simulink library "simpower_extensions_1"  (Simulink 7.4)
settings: Solver=ode45  SolverMode=SingleTasking  StartTime=0.0  StopTime=10.0  RelTol=1e-3
values from neighbouring files (symbols this model uses):
  Av = 10^(Gdb/20)    (= 6.3095734448)    [series_shunt_2c.m]
undefined symbols (not defined in the file or in its folder): f1, f2, Fs, get, magnitude, One, sided, Two
libraries: powerlib x71, dspindex x36, dsparch4 x22, dspsigops x18, dspbuff3 x12, dspxfrm3 x12, dsparch3 x12, dspsnks4 x6, dspmtrx3 x6, simpower_extensions_1 x1, simulink x1, simulink_extras x1
(part 1 of 3)
settings Model: Creator=Dick Benson  LastModifiedBy=Dick  ModifiedHistory=1st cut at EE circuit library.

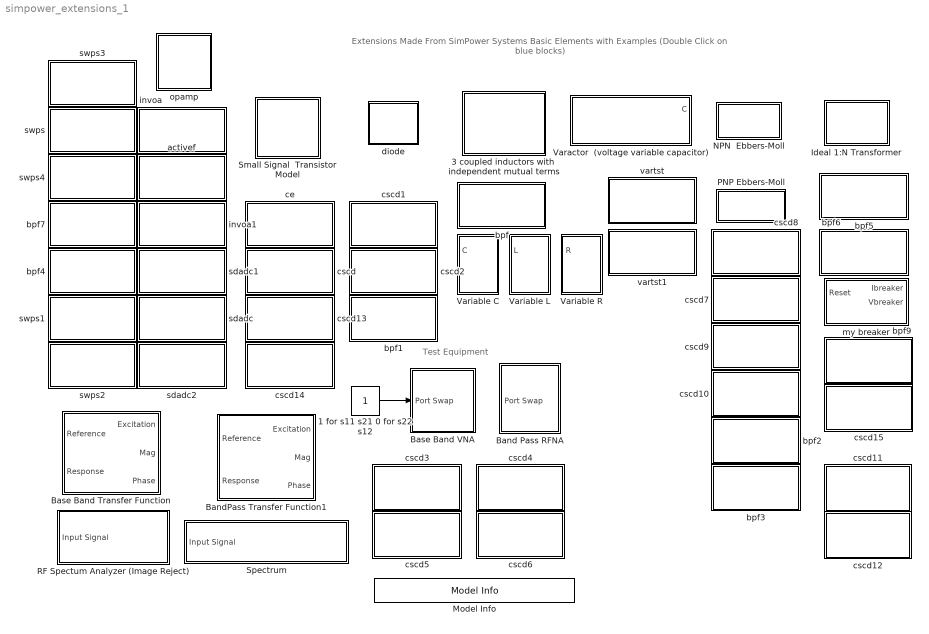
== system simpower_extensions_1 ==
  note: Extensions Made From SimPower Systems Basic Elements
      | with Examples (Double Click on blue blocks)
  note: Test Equipment
  1 for s11 s21 0 for s22 s12 : Constant  OutDataType=fixdt(1, 16)  OutScaling=2^0
  3 coupled inductors with  independent mutual terms : Subsystem  mask{L1=1e-6, L2=1e-6, L3=1e-6, M12=0.1e-6, M23=0.1e-6, M13=1e-8}
      mask prompts: L1 "L1="; L2 "L2="; L3 "L3="; M12 "M12="; M23 "M23="; M13 "M13="
  Band Pass RFNA : Subsystem  Description=Spectrum Analyzer  mask{Fc=75e6, BW=20e6, Frame_Size=512}
      mask prompts: Fc "Center Freq"; BW "Bandwidth"; Frame_Size "FFT SIze (256,512,1024 etc)"
  BandPass Transfer Function1 : Subsystem  Description=Spectrum Analyzer  mask{BW=40e6, Fc=100e6, NFFT=1024, Avg_fac=100}
      mask prompts: BW "Bandwidth"; Fc "Center Freq"; NFFT "FFT Length (power of 2)"; Avg_fac "Averaging Factor (>=1)"
  Base Band Transfer Function : Subsystem  Description=Spectrum Analyzer  mask{BW=100e6, NFFT=1024, Avg_fac=100}
      mask prompts: BW "Bandwidth"; NFFT "FFT Length (power of 2)"; Avg_fac "Averaging Factor (>=1)"
  Base Band VNA : Subsystem  Description=Spectrum Analyzer  mask{BW=2e8, Frame_Size=512}
      mask prompts: BW "Bandwidth"; Frame_Size "FFT SIze (256,512,1024 etc)"
  Ideal 1:N Transformer : Subsystem  mask{N=10}
      mask prompts: N "Turns Ratio Secondary/Primary"
  Model Info : simulink/Model-Wide Utilities/Model Info  SystemSampleTime=-1  InitialBlockCM=None  BlockCM=None  Frame=on  DisplayStringWithTags=Copywrite 2005-2011 The MathWorks, Inc.  HorizontalTextAlignment=Center  LeftAlignmentValue=0.5  SourceBlockDiagram=simpower_extensions_1  TagMaxNumber=20
  "NPN  Ebbers-Moll " : Subsystem  mask{Beta=100, IEs=1e-8;, ICs=1e-8;, Ro=1e5, Cbc=5e-12, Cbe=50e-12, Rbb=100}
      mask init:
      | k = 1.38e-23;
      | q = 1.6e-19;
      | T = 290;
      | Vt = k*T/q;
  PNP Ebbers-Moll : Subsystem  mask{Beta=100, IEs=1e-8;, ICs=1e-8;, Ro=1e5, Cbc=5e-12, Cbe=50e-12, Rbb=100}
      mask init:
      | k = 1.38e-23;
      | q = 1.6e-19;
      | T = 290;
      | Vt = k*T/q;
  RF Spectum Analyzer (Image Reject) : Subsystem  Description=Spectrum Analyzer  mask{BW=.2e6, Fc=1e6, Zo=50}
      mask prompts: BW "Bandwidth"; Fc "Center Freq"; Zo "Load Resistance"
      mask Display: fprintf('Spectrum Analyzer \n Fc=%7.2f MHz \n BW=%7.2f MHz',Fc/1e6,BW/1e6)
  Small Signal  Transistor Model : Subsystem  mask{Rbc=1e5, Cbc=1.5e-12, gm=0.5, Rbe=1000, Cbe=50e-12, Rbb=100}
      mask Display: disp('transistor')
  Spectrum : Subsystem  Description=Spectrum Analyzer  mask{BW=1e6, Zo=50}
      mask prompts: BW "Bandwidth"; Zo "Load Zo"
      mask Display: fprintf('Baseband Spectrum Analyzer \n  BW=%7.2f MHz', BW/1e6)
  Varactor  (voltage variable capacitor) : Subsystem  mask{Cjo=100e-12, Vj=0.7, M=0.5, Cp=5e-12}
      mask prompts: Cjo "Capacitance Vr==0 (Cjo)"; Vj "Junction Potential (Vj)"; M "Grading Coefficient (M)"; Cp "Package Capacitance (Cp)"
      mask Display: disp('C = Cp + Cjo/((1+Vr/Vj)^M)')
  Variable C : Subsystem
  Variable L : Subsystem
  Variable R : Subsystem
  activef : Subsystem
      settings: OpenFcn=rauch_c
      mask Display: disp('Active Filter');
  bpf : Subsystem
      settings: OpenFcn=coupled_inductor_test
      mask Display: disp('Bandpass Filter');
  bpf1 : Subsystem
      settings: OpenFcn=cl_e_5x
      mask Display: disp('Class E RF Amp');
  bpf2 : Subsystem
      settings: OpenFcn=norton_5_nl_push_pull
      mask Display: disp('Push Pull \nNorton Amp');
  bpf3 : Subsystem
      settings: OpenFcn=series_shunt_2a; edit series_shunt_2c;
      mask Display: disp('Push Pull \nSeries-Shunt Amp');
  bpf4 : Subsystem
      settings: OpenFcn=DC_2_AC_1
      mask Display: disp('DC_2_AC');
  bpf5 : Subsystem
      settings: OpenFcn=transformer_1
      mask Display: disp('Transformer Test');
  bpf6 : Subsystem
      settings: OpenFcn=transformer_2
      mask Display: disp('Transformer \nModeling');
  bpf7 : Subsystem
      settings: OpenFcn=sepic_2
      mask Display: disp('SEPIC');
  bpf9 : Subsystem
      settings: OpenFcn=circuitbreaker_1
      mask Display: disp('Breaker Test');
  ce : Subsystem
      settings: OpenFcn=xistor_1
      mask Display: disp('Common Emitter');
  cscd : Subsystem
      settings: OpenFcn=xistor_2
      mask Display: disp('Cascode');
  cscd1 : Subsystem
      settings: OpenFcn=diode_3
      mask Display: disp('Diode Test');
  cscd10 : Subsystem
      settings: OpenFcn=ebbers_moll_3;
      mask Display: disp('Discrete\n Op Amp');
  cscd11 : Subsystem
      settings: OpenFcn=trans_line_1
      mask Display: disp('Distributed \nTransmission \nLine');
  cscd12 : Subsystem
      settings: OpenFcn=trans_line_2
      mask Display: disp('Distributed \nTransmission \n Balanced Line');
  cscd13 : Subsystem
      settings: OpenFcn=super_regen_1;
      mask Display: disp('Super Regen I');
  cscd14 : Subsystem
      settings: OpenFcn=super_regen_2;
      mask Display: disp('Super Regen II');
  cscd15 : Subsystem
      settings: OpenFcn=tripler_sps_4
      mask Display: disp('Diode \nVoltage Tripler');
  cscd2 : Subsystem
      settings: OpenFcn=mix_1
      mask Display: disp('Diode Ring Mixer');
  cscd3 : Subsystem
      settings: OpenFcn=base_band_spar
      mask Display: disp('Base Band RFNA');
  cscd4 : Subsystem
      settings: OpenFcn=band_pass_spar
      mask Display: disp('Band Pass RFNA');
  cscd5 : Subsystem
      settings: OpenFcn=c6_p8x
      mask Display: disp('Lumped Xmission \nLine');
  cscd6 : Subsystem
      settings: OpenFcn=pi_match_1
      mask Display: disp('Pi Net Z Match');
  cscd7 : Subsystem
      settings: OpenFcn=osc_2
      mask Display: disp('Oscillator');
  cscd8 : Subsystem
      settings: OpenFcn=ebbers_moll_1
      mask Display: disp('Curve Trace');
  cscd9 : Subsystem
      settings: OpenFcn=ebbers_moll_2;
      mask Display: disp('Diff Pair');
  diode : Subsystem  mask{Is=1e-8, Rfwd=1}
      mask prompts: Is "Saturation Current"; Rfwd "Forward Resistance"
      mask Display: plot(-140,-140,150,140,2*[30,30,59,30,30,0]-75,(2*[71,50,72,92,71,71]-92),2*[59,59]-75,(2*[50,93]-92),[116,59]-16,(2*[71,71]-90));
  invoa : Subsystem
      settings: OpenFcn=op_amp
      mask Display: disp('Inverting Op Amp');
  invoa1 : Subsystem
      settings: OpenFcn=linear_reg_2
      mask Display: disp('Linear Regulators');
  my breaker : Subsystem  mask{Iset=10, Tau=.1}
      mask prompts: Iset "Current Rating (Amps)"; Tau "Mechanical Time Constant (Sec)"
  opamp : Subsystem  mask{f2=f2, f1=f1, Av=Av, v_min=-3, v_max=3, slew_rate=2e9}
      mask prompts: f2 "break freq 2 in Hz"; f1 "break freq 1 in Hz"; Av "Av (voltage gain)"; v_min "Min Output"; v_max "Max Output"; slew_rate "slew rate (v/s)"
      mask Display: plot([0 1 0 0] , [1 0 -1 1 ]); text(0.15,0.4,'+'); text(0.15,-0.4,'-');
  sdadc : Subsystem
      settings: OpenFcn=constant_gain_variable_Q
      mask Display: disp('Variable Q');
  sdadc1 : Subsystem
      settings: OpenFcn=sigma2nd_d
      mask Display: disp('Sigma Delta ADC');
  sdadc2 : Subsystem
      settings: OpenFcn=Led_photo_transZ_3;
      mask Display: disp('LED - PhotoDiode');
  swps : Subsystem
      settings: OpenFcn=swps_2
      mask Display: disp('Switching PS \n (Buck)');
  swps1 : Subsystem
      settings: OpenFcn=pwr_amp_1
      mask Display: disp('Switching \n Audio Amp');
  swps2 : Subsystem
      settings: OpenFcn=pwr_amp_2
      mask Display: disp('Switching Bridge \n Audio Amp');
  swps3 : Subsystem
      settings: OpenFcn=swps_3
      mask Display: disp('Switching PS \n (Flyback)');
  swps4 : Subsystem
      settings: OpenFcn=dc2dc_boost_3
      mask Display: disp('Switching PS \n (Boost)');
  vartst : Subsystem
      settings: OpenFcn=varactor_test
      mask Display: disp('Varactor Test');
  vartst1 : Subsystem
      settings: OpenFcn=vco_2
      mask Display: disp('VCO with Varactor');
  wires:
  1 for s11 s21 0 for s22 s12/1 -> Base Band VNA/1(Port Swap)

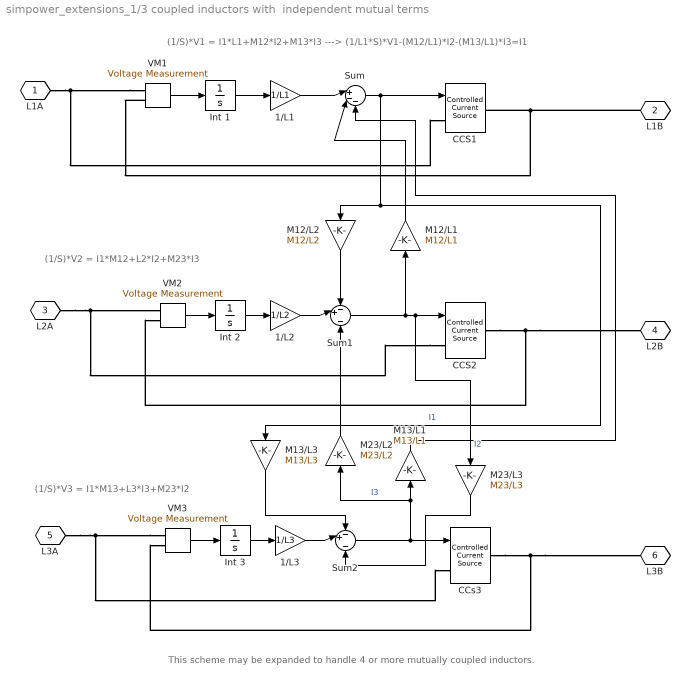
== system simpower_extensions_1/3 coupled inductors with  independent mutual terms ==
  note: This scheme may be expanded to handle 4 or more mutually coupled inductors.
  note: (1/S)*V3 = I1*M13+L3*I3+M23*I2
  note: (1/S)*V2 = I1*M12+L2*I2+M23*I3
  note: (1/S)*V1 = I1*L1+M12*I2+M13*I3 ---> (1/L1*S)*V1-(M12/L1)*I2-(M13/L1)*I3=I1
  1/L1 : Gain  Gain=1/L1  ParameterDataType=sfix(16)  ParameterScaling=2^0  OutDataType=sfix(16)  OutScaling=2^0  SaturateOnIntegerOverflow=on  OutDataTypeStr=Inherit: Same as input  ParamDataTypeStr=Inherit: Same as input
  1/L2 : Gain  Gain=1/L2  ParameterDataType=sfix(16)  ParameterScaling=2^0  OutDataType=sfix(16)  OutScaling=2^0  SaturateOnIntegerOverflow=on  OutDataTypeStr=Inherit: Same as input  ParamDataTypeStr=Inherit: Same as input
  1/L3 : Gain  Gain=1/L3  ParameterDataType=sfix(16)  ParameterScaling=2^0  OutDataType=sfix(16)  OutScaling=2^0  SaturateOnIntegerOverflow=on  OutDataTypeStr=Inherit: Same as input  ParamDataTypeStr=Inherit: Same as input
  CCS1 : powerlib/Electrical Sources/Controlled Current Source  Description=source block  DialogController=POWERSYS.PowerSysDialog  SystemSampleTime=-1  Initialize=off  Source_Type=AC  Amplitude=0  Phase=0  Frequency=0  Measurements=None
      settings: AttributesFormatString=\n
  CCS2 : powerlib/Electrical Sources/Controlled Current Source  Description=source block  DialogController=POWERSYS.PowerSysDialog  SystemSampleTime=-1  Initialize=off  Source_Type=AC  Amplitude=0  Phase=0  Frequency=0  Measurements=None
      settings: AttributesFormatString=\n
  CCs3 : powerlib/Electrical Sources/Controlled Current Source  Description=source block  DialogController=POWERSYS.PowerSysDialog  SystemSampleTime=-1  Initialize=off  Source_Type=AC  Amplitude=0  Phase=0  Frequency=0  Measurements=None
      settings: AttributesFormatString=\n
  Int 1 : Integrator
  Int 2 : Integrator
  Int 3 : Integrator
  M12/L1 : Gain  Gain=M12/L1  ParameterDataType=sfix(16)  ParameterScaling=2^0  OutDataType=sfix(16)  OutScaling=2^0  SaturateOnIntegerOverflow=on  OutDataTypeStr=Inherit: Same as input  ParamDataTypeStr=Inherit: Same as input
  M12/L2 : Gain  Gain=M12/L2  ParameterDataType=sfix(16)  ParameterScaling=2^0  OutDataType=sfix(16)  OutScaling=2^0  SaturateOnIntegerOverflow=on  OutDataTypeStr=Inherit: Same as input  ParamDataTypeStr=Inherit: Same as input
  M13/L1 : Gain  Gain=M13/L1  ParameterDataType=sfix(16)  ParameterScaling=2^0  OutDataType=sfix(16)  OutScaling=2^0  SaturateOnIntegerOverflow=on  OutDataTypeStr=Inherit: Same as input  ParamDataTypeStr=Inherit: Same as input
  M13/L3 : Gain  Gain=M13/L3  ParameterDataType=sfix(16)  ParameterScaling=2^0  OutDataType=sfix(16)  OutScaling=2^0  SaturateOnIntegerOverflow=on  OutDataTypeStr=Inherit: Same as input  ParamDataTypeStr=Inherit: Same as input
  M23/L2 : Gain  Gain=M23/L2  ParameterDataType=sfix(16)  ParameterScaling=2^0  OutDataType=sfix(16)  OutScaling=2^0  SaturateOnIntegerOverflow=on  OutDataTypeStr=Inherit: Same as input  ParamDataTypeStr=Inherit: Same as input
  M23/L3 : Gain  Gain=M23/L3  ParameterDataType=sfix(16)  ParameterScaling=2^0  OutDataType=sfix(16)  OutScaling=2^0  SaturateOnIntegerOverflow=on  OutDataTypeStr=Inherit: Same as input  ParamDataTypeStr=Inherit: Same as input
  Sum : Sum  Inputs=|+--  OutDataType=sfix(16)  OutScaling=2^0  SaturateOnIntegerOverflow=on
  Sum1 : Sum  Inputs=-+|-  OutDataType=sfix(16)  OutScaling=2^0  SaturateOnIntegerOverflow=on
  Sum2 : Sum  Inputs=-+|-  OutDataType=sfix(16)  OutScaling=2^0  SaturateOnIntegerOverflow=on
  VM1 : powerlib/Measurements/Voltage Measurement  Tag=PoWeRsYsTeMmEaSuReMeNt  DialogController=POWERSYS.PowerSysDialog  SystemSampleTime=-1  PhasorSimulation=off  OutputType=Magnitude  PSBequivalent=0
  VM2 : powerlib/Measurements/Voltage Measurement  Tag=PoWeRsYsTeMmEaSuReMeNt  DialogController=POWERSYS.PowerSysDialog  SystemSampleTime=-1  PhasorSimulation=off  OutputType=Magnitude  PSBequivalent=0
  VM3 : powerlib/Measurements/Voltage Measurement  Tag=PoWeRsYsTeMmEaSuReMeNt  DialogController=POWERSYS.PowerSysDialog  SystemSampleTime=-1  PhasorSimulation=off  OutputType=Magnitude  PSBequivalent=0
  L1A : PMIOPort  Tag=PMCPort  Port=1  Side=Left
  L1B : PMIOPort  Tag=PMCPort  Port=2  Side=Right
  L2A : PMIOPort  Tag=PMCPort  Port=3  Side=Left
  L2B : PMIOPort  Tag=PMCPort  Port=4  Side=Right
  L3A : PMIOPort  Tag=PMCPort  Port=5  Side=Left
  L3B : PMIOPort  Tag=PMCPort  Port=6  Side=Right
  wires:
  M23/L3/1 -> Sum2/3
  M13/L3/1 -> Sum2/1
  M23/L2/1 -> Sum1/3
  M13/L1/1 -> Sum/3
  1/L3/1 -> Sum2/2
  Sum2/1 -> M23/L2/1, M13/L1/1, CCs3/1  "I3"
  VM3/1 -> Int 3/1
  Int 3/1 -> 1/L3/1
  M12/L2/1 -> Sum1/1
  M12/L1/1 -> Sum/2
  1/L2/1 -> Sum1/2
  Sum1/1 -> M23/L3/1, CCS2/1, M12/L1/1  "I2"
  Sum/1 -> M13/L3/1, M12/L2/1, CCS1/1  "I1"
  1/L1/1 -> Sum/1
  VM2/1 -> Int 2/1
  Int 2/1 -> 1/L2/1
  VM1/1 -> Int 1/1
  Int 1/1 -> 1/L1/1
  connections:
  CCs3/RConn1 -- L3B/RConn1 -- VM3/LConn2
  VM3/LConn1 -- L3A/RConn1 -- CCs3/LConn1
  VM2/LConn2 -- CCS2/RConn1 -- L2B/RConn1
  CCS2/LConn1 -- VM2/LConn1 -- L2A/RConn1
  VM1/LConn2 -- L1B/RConn1 -- CCS1/RConn1
  VM1/LConn1 -- CCS1/LConn1 -- L1A/RConn1

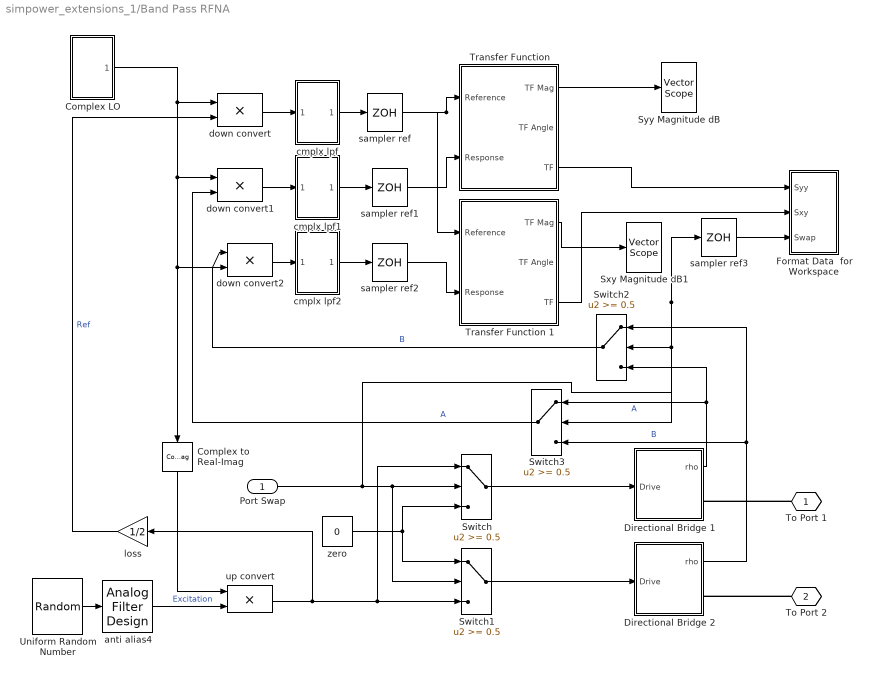
== system simpower_extensions_1/Band Pass RFNA ==
  Port Swap : Inport  OutDataType=sfix(16)  OutScaling=2^0
  Complex LO : Subsystem
  Complex to Real-Imag : ComplexToRealImag  Output=Real
  Directional Bridge 1 : Subsystem  mask{Zo=50}
      mask prompts: Zo "Zo="
  Directional Bridge 2 : Subsystem  mask{Zo=50}
      mask prompts: Zo "Zo="
  Format Data  for Workspace : Subsystem
  Switch{,1..3} (4 alike) : Switch  Threshold=0.5  SaturateOnIntegerOverflow=on
  Sxy Magnitude dB1 : dspsnks4/Vector Scope  DialogController=dspdialog.VectorScope  DialogControllerArgs=DataTag0  ScopeProperties=on  Domain=Frequency  HorizSpan=1  DisplayProperties=off  AxisGrid=on  Memory=off  FrameNumber=on  AxisLegend=off  AxisZoom=off  OpenScopeAtSimStart=on  OpenScopeImmediately=off  FigPos=[78 403 372 236]  AxisProperties=off  XUnits=Hertz  XRange=[-Fs/2...Fs/2]  InheritXIncr=off  XIncr=1/(1.28*BW)  XLabel=Time  XLimit=Auto  XMin=0  XMax=1  XStart=0  YUnits=dB  YLabel=dB  LineProperties=off  LineColors=[1 0 0]|[1 0 0]  XAxisParamsVer=6.9
      settings: YMin=-50.7136770041669  YMax=0.738454215323831
  Syy Magnitude dB : dspsnks4/Vector Scope  DialogController=dspdialog.VectorScope  DialogControllerArgs=DataTag1  ScopeProperties=on  Domain=Frequency  HorizSpan=1  DisplayProperties=off  AxisGrid=on  Memory=off  FrameNumber=on  AxisLegend=off  AxisZoom=off  OpenScopeAtSimStart=on  OpenScopeImmediately=off  FigPos=[79 118 372 236]  AxisProperties=off  XUnits=Hertz  XRange=[-Fs/2...Fs/2]  InheritXIncr=off  XIncr=1/(1.28*BW)  XLabel=Time  XLimit=Auto  XMin=0  XMax=1  XStart=0  YUnits=dB  YLabel=dB  LineProperties=off  LineColors=[1 0 0]|[1 0 0]  XAxisParamsVer=6.9
      settings: YMin=-22.5936403056033  YMax=0.0324469649011859
  "Transfer Function " : Subsystem  mask{NFFT=Frame_Size, Navg=100, pcnt=100, unwrap_flag=on}
      mask prompts: NFFT "FFT length (power of 2):"; Navg "Spectral Averaging Factor (>=1):"; pcnt "Percentage of  Alias Free Data  (<=100)"; unwrap_flag "Unwrap Phase"
      mask Display: disp('Transfer Function \n Estimation (v2.0) ')
  Transfer Function 1 : Subsystem  mask{NFFT=Frame_Size, Navg=100, pcnt=100, unwrap_flag=on}
      mask prompts: NFFT "FFT length (power of 2):"; Navg "Spectral Averaging Factor (>=1):"; pcnt "Percentage of  Alias Free Data  (<=100)"; unwrap_flag "Unwrap Phase"
      mask Display: disp('Transfer Function \n Estimation (v2.0) ')
  Uniform Random Number : UniformRandomNumber  SampleTime=1/(2.56*BW)
  anti alias4 : dsparch4/Analog Filter Design  method=Elliptic  filttype=Lowpass  N=8  Wlo=BW*pi  Whi=80  Rp=2  Rs=100
  cmplx lpf : Subsystem
  cmplx lpf1 : Subsystem
  cmplx lpf2 : Subsystem
  down convert : Product  OutDataType=sfix(16)  OutScaling=2^0  SaturateOnIntegerOverflow=on  InputSameDT=on  OutDataTypeStr=Inherit: Same as first input
  down convert1 : Product  OutDataType=sfix(16)  OutScaling=2^0  SaturateOnIntegerOverflow=on  InputSameDT=on  OutDataTypeStr=Inherit: Same as first input
  down convert2 : Product  OutDataType=sfix(16)  OutScaling=2^0  SaturateOnIntegerOverflow=on  InputSameDT=on  OutDataTypeStr=Inherit: Same as first input
  loss : Gain  Gain=1/2  ParameterDataType=sfix(16)  ParameterScaling=2^0  OutDataType=sfix(16)  OutScaling=2^0  SaturateOnIntegerOverflow=on  OutDataTypeStr=Inherit: Same as input  ParamDataTypeStr=Inherit: Same as input
  sampler ref : ZeroOrderHold  SampleTime=1/(1.28*BW)
  sampler ref1 : ZeroOrderHold  SampleTime=1/(1.28*BW)
  sampler ref2 : ZeroOrderHold  SampleTime=1/(1.28*BW)
  sampler ref3 : ZeroOrderHold  SampleTime=256/(1.28*BW)
  up convert : Product  OutDataType=sfix(16)  OutScaling=2^0  SaturateOnIntegerOverflow=on  InputSameDT=on  OutDataTypeStr=Inherit: Same as first input
  zero : Constant  Value=0  OutDataType=sfix(16)  OutScaling=2^0
  To Port 1 : PMIOPort  Tag=PMCPort  Port=1  Side=Right
  To Port 2 : PMIOPort  Tag=PMCPort  Port=2  Side=Right
  wires:
  sampler ref3/1 -> Format Data  for Workspace/3(Swap)
  Transfer Function 1/1(TF Mag) -> Sxy Magnitude dB1/1
  "Transfer Function "/1(TF Mag) -> Syy Magnitude dB/1
  "Transfer Function "/3("TF ") -> Format Data  for Workspace/1(Syy)
  Directional Bridge 2/1(rho) -> Switch2/1, Switch3/3  "B"
  Directional Bridge 1/1(rho) -> Switch3/1, Switch2/3  "A"
  Switch2/1 -> down convert2/2  "B"
  Switch3/1 -> down convert1/2  "A"
  Complex to Real-Imag/1 -> up convert/1
  up convert/1 -> loss/1, Switch/1, Switch1/3
  anti alias4/1 -> up convert/2  "Excitation"
  sampler ref2/1 -> Transfer Function 1/2(Response)
  cmplx lpf2/1(Out1) -> sampler ref2/1
  down convert2/1 -> cmplx lpf2/1(In1)
  sampler ref1/1 -> "Transfer Function "/2(Response)
  cmplx lpf1/1(Out1) -> sampler ref1/1
  down convert1/1 -> cmplx lpf1/1(In1)
  cmplx lpf/1(Out1) -> sampler ref/1
  down convert/1 -> cmplx lpf/1(In1)
  Complex LO/1(cos/sin) -> Complex to Real-Imag/1, down convert2/1, down convert1/1, down convert/1
  sampler ref/1 -> Transfer Function 1/1(Reference), "Transfer Function "/1(Reference)
  Uniform Random Number/1 -> anti alias4/1
  Transfer Function 1/3("TF ") -> Format Data  for Workspace/2(Sxy)
  Switch1/1 -> Directional Bridge 2/1(Drive)
  Switch/1 -> Directional Bridge 1/1(Drive)
  loss/1 -> down convert/2  "Ref"
  Port Swap/1 -> sampler ref3/1, Switch3/2, Switch2/2, Switch/2, Switch1/2
  zero/1 -> Switch1/1, Switch/3
  connections:
  To Port 2/RConn1 -- Directional Bridge 2/RConn1
  To Port 1/RConn1 -- Directional Bridge 1/RConn1

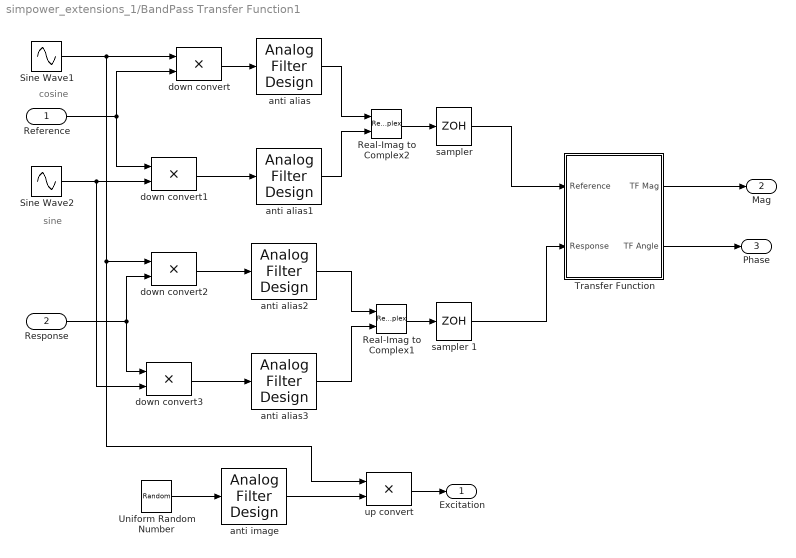
== system simpower_extensions_1/BandPass Transfer Function1 ==
  note: cosine
  note: sine
  Reference : Inport  OutDataType=sfix(16)  OutScaling=2^0
  Response : Inport  Port=2  OutDataType=sfix(16)  OutScaling=2^0
  Real-Imag to Complex1 : RealImagToComplex
  Real-Imag to Complex2 : RealImagToComplex
  Sine Wave1 : Sin  Amplitude=1  Bias=0  Frequency=2*pi*(Fc)  Phase=-pi/2  Samples=10  SampleTime=0  Offset=0
  Sine Wave2 : Sin  Amplitude=1  Bias=0  Frequency=2*pi*(Fc)  Phase=0  Samples=10  SampleTime=0  Offset=0
  "Transfer Function " : Subsystem  mask{NFFT=NFFT, Navg=Avg_fac, pcnt=100/1.28, unwrap_flag=on}
      mask prompts: NFFT "FFT length (power of 2):"; Navg "Spectral Averaging Factor (>=1):"; pcnt "Percentage of  Alias Free Data  (<=100)"; unwrap_flag "Unwrap Phase"
      mask Display: disp('Transfer Function \n Estimation (v2.0) ')
  Uniform Random Number : UniformRandomNumber  SampleTime=1/(2.56*BW)
  anti alias{,1..3} (4 alike) : dsparch4/Analog Filter Design  method=Elliptic  filttype=Lowpass  N=8  Wlo=BW*pi  Whi=80  Rp=2  Rs=100
  anti image : dsparch4/Analog Filter Design  method=Elliptic  filttype=Lowpass  N=9  Wlo=BW*pi  Whi=80  Rp=2  Rs=100
  down convert{,1..3} (4 alike) : Product  OutDataType=sfix(16)  OutScaling=2^0  SaturateOnIntegerOverflow=on  InputSameDT=on  OutDataTypeStr=Inherit: Same as first input
  "sampler " : ZeroOrderHold  SampleTime=1/(1.28*BW)
  sampler 1 : ZeroOrderHold  SampleTime=1/(1.28*BW)
  up convert : Product  OutDataType=sfix(16)  OutScaling=2^0  SaturateOnIntegerOverflow=on  InputSameDT=on  OutDataTypeStr=Inherit: Same as first input
  Excitation : Outport  OutDataType=sfix(16)  OutScaling=2^0
  Mag : Outport  Port=2  OutDataType=sfix(16)  OutScaling=2^0
  Phase : Outport  Port=3  OutDataType=sfix(16)  OutScaling=2^0
  wires:
  Reference/1 -> down convert/2, down convert1/1
  down convert/1 -> anti alias/1
  Sine Wave1/1 -> down convert/1, down convert2/1, up convert/1
  Sine Wave2/1 -> down convert1/2, down convert3/2
  Response/1 -> down convert3/1, down convert2/2
  down convert2/1 -> anti alias2/1
  anti alias2/1 -> Real-Imag to Complex1/1
  anti alias3/1 -> Real-Imag to Complex1/2
  down convert3/1 -> anti alias3/1
  Real-Imag to Complex1/1 -> sampler 1/1
  Uniform Random Number/1 -> anti image/1
  up convert/1 -> Excitation/1
  "Transfer Function "/1(TF Mag) -> Mag/1
  "Transfer Function "/2(TF Angle) -> Phase/1
  anti alias/1 -> Real-Imag to Complex2/1
  anti alias1/1 -> Real-Imag to Complex2/2
  Real-Imag to Complex2/1 -> "sampler "/1
  "sampler "/1 -> "Transfer Function "/1(Reference)
  sampler 1/1 -> "Transfer Function "/2(Response)
  down convert1/1 -> anti alias1/1
  anti image/1 -> up convert/2

== system simpower_extensions_1/Base Band Transfer Function ==
  note: Bandlimited Excitation
  "Reference " : Inport  OutDataType=sfix(16)  OutScaling=2^0
  Response : Inport  Port=2  OutDataType=sfix(16)  OutScaling=2^0
  "Transfer Function " : Subsystem  mask{NFFT=NFFT, Navg=Avg_fac, pcnt=100/1.28, unwrap_flag=on}
      mask prompts: NFFT "FFT length (power of 2):"; Navg "Spectral Averaging Factor (>=1):"; pcnt "Percentage of  Alias Free Data  (<=100)"; unwrap_flag "Unwrap Phase"
      mask Display: disp('Transfer Function \n Estimation (v2.0) ')
  Uniform Random Number : UniformRandomNumber  SampleTime=1/(2.56*BW)
  anti alias : dsparch4/Analog Filter Design  method=Elliptic  filttype=Lowpass  N=8  Wlo=BW*2*pi  Whi=80  Rp=2  Rs=100
  anti alias1 : dsparch4/Analog Filter Design  method=Elliptic  filttype=Lowpass  N=8  Wlo=BW*2*pi  Whi=80  Rp=2  Rs=100
  anti alias2 : dsparch4/Analog Filter Design  method=Elliptic  filttype=Lowpass  N=8  Wlo=BW*2*pi  Whi=80  Rp=2  Rs=100
  sampler : ZeroOrderHold  SampleTime=1/(2.56*BW)
  sampler1 : ZeroOrderHold  SampleTime=1/(2.56*BW)
  Excitation : Outport  OutDataType=sfix(16)  OutScaling=2^0
  Mag : Outport  Port=2  OutDataType=sfix(16)  OutScaling=2^0
  Phase : Outport  Port=3  OutDataType=sfix(16)  OutScaling=2^0
  wires:
  anti alias/1 -> sampler/1
  "Reference "/1 -> anti alias/1
  anti alias1/1 -> sampler1/1
  Response/1 -> anti alias1/1
  Uniform Random Number/1 -> anti alias2/1
  anti alias2/1 -> Excitation/1
  sampler/1 -> "Transfer Function "/1(Reference)
  sampler1/1 -> "Transfer Function "/2(Response)
  "Transfer Function "/1(TF Mag) -> Mag/1
  "Transfer Function "/2(TF Angle) -> Phase/1

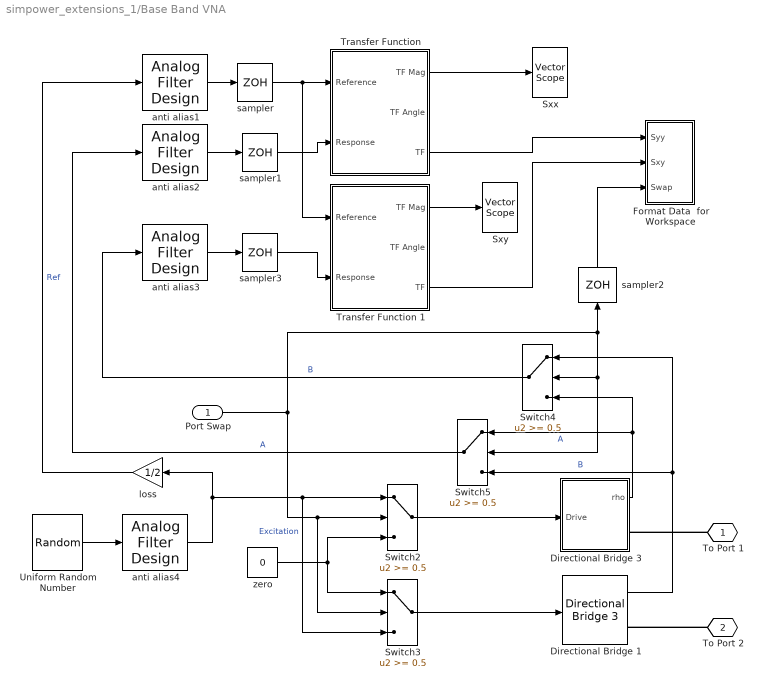
== system simpower_extensions_1/Base Band VNA ==
  Port Swap : Inport  OutDataType=sfix(16)  OutScaling=2^0
  Directional Bridge 1 : simpower_extensions_1/Base Band VNA/Directional Bridge 3  SystemSampleTime=-1  Zo=50
  Directional Bridge 3 : Subsystem  mask{Zo=50}
      mask prompts: Zo "Zo="
  Format Data  for Workspace : Subsystem
  Switch{2..5} (4 alike) : Switch  Threshold=0.5  SaturateOnIntegerOverflow=on
  Sxx : dspsnks4/Vector Scope  DialogController=dspdialog.VectorScope  DialogControllerArgs=DataTag22  ScopeProperties=on  Domain=Frequency  HorizSpan=1  DisplayProperties=off  AxisGrid=on  Memory=off  FrameNumber=on  AxisLegend=off  AxisZoom=off  OpenScopeAtSimStart=on  OpenScopeImmediately=off  FigPos=get(0,'defaultfigureposition')  AxisProperties=off  XUnits=Hertz  XRange=[0...Fs/2]  InheritXIncr=off  XIncr=1/(2.56*BW)  XLabel=Time  XLimit=Auto  XMin=0  XMax=1  XStart=0  YUnits=dB  YLabel=Amplitude  LineProperties=off  XAxisParamsVer=6.9
      settings: YMin=-30  YMax=25
  Sxy : dspsnks4/Vector Scope  DialogController=dspdialog.VectorScope  DialogControllerArgs=DataTag23  ScopeProperties=on  Domain=Frequency  HorizSpan=1  DisplayProperties=off  AxisGrid=on  Memory=off  FrameNumber=on  AxisLegend=off  AxisZoom=off  OpenScopeAtSimStart=on  OpenScopeImmediately=off  FigPos=get(0,'defaultfigureposition')  AxisProperties=off  XUnits=Hertz  XRange=[0...Fs/2]  InheritXIncr=off  XIncr=1/(2.56*BW)  XLabel=Time  XLimit=Auto  XMin=0  XMax=1  XStart=0  YUnits=dB  YLabel=Amplitude  LineProperties=off  XAxisParamsVer=6.9
      settings: YMin=-30  YMax=25
  "Transfer Function " : Subsystem  mask{NFFT=Frame_Size, Navg=100, pcnt=100, unwrap_flag=on}
      mask prompts: NFFT "FFT length (power of 2):"; Navg "Spectral Averaging Factor (>=1):"; pcnt "Percentage of  Alias Free Data  (<=100)"; unwrap_flag "Unwrap Phase"
      mask Display: disp('Transfer Function \n Estimation (v2.0) ')
  Transfer Function 1 : Subsystem  mask{NFFT=Frame_Size, Navg=100, pcnt=100, unwrap_flag=on}
      mask prompts: NFFT "FFT length (power of 2):"; Navg "Spectral Averaging Factor (>=1):"; pcnt "Percentage of  Alias Free Data  (<=100)"; unwrap_flag "Unwrap Phase"
      mask Display: disp('Transfer Function \n Estimation (v2.0) ')
  Uniform Random Number : UniformRandomNumber  SampleTime=1/(2.56*BW)
  anti alias{1..4} (4 alike) : dsparch4/Analog Filter Design  method=Elliptic  filttype=Lowpass  N=8  Wlo=BW*2*pi  Whi=80  Rp=2  Rs=100
  loss : Gain  Gain=1/2  ParameterDataType=sfix(16)  ParameterScaling=2^0  OutDataType=sfix(16)  OutScaling=2^0  SaturateOnIntegerOverflow=on  OutDataTypeStr=Inherit: Same as input  ParamDataTypeStr=Inherit: Same as input
  sampler : ZeroOrderHold  SampleTime=1/(2.56*BW)
  sampler1 : ZeroOrderHold  SampleTime=1/(2.56*BW)
  sampler2 : ZeroOrderHold  SampleTime=256/(2.56*BW)
  sampler3 : ZeroOrderHold  SampleTime=1/(2.56*BW)
  zero : Constant  Value=0  OutDataType=sfix(16)  OutScaling=2^0
  To Port 1 : PMIOPort  Tag=PMCPort  Port=1  Side=Right
  To Port 2 : PMIOPort  Tag=PMCPort  Port=2  Side=Right
  wires:
  sampler/1 -> "Transfer Function "/1(Reference), Transfer Function 1/1(Reference)
  anti alias1/1 -> sampler/1
  anti alias2/1 -> sampler1/1
  Uniform Random Number/1 -> anti alias4/1
  anti alias3/1 -> sampler3/1
  sampler3/1 -> Transfer Function 1/2(Response)
  anti alias4/1 -> loss/1, Switch3/3, Switch2/1  "Excitation"
  loss/1 -> anti alias1/1  "Ref"
  Port Swap/1 -> Switch3/2, Switch2/2, Switch4/2, Switch5/2, sampler2/1
  zero/1 -> Switch2/3, Switch3/1
  Switch2/1 -> Directional Bridge 3/1(Drive)
  Switch3/1 -> Directional Bridge 1/1
  Switch5/1 -> anti alias2/1  "A"
  Switch4/1 -> anti alias3/1  "B"
  Directional Bridge 3/1(rho) -> Switch4/3, Switch5/1  "A"
  Directional Bridge 1/1 -> Switch5/3, Switch4/1  "B"
  sampler1/1 -> "Transfer Function "/2(Response)
  "Transfer Function "/1(TF Mag) -> Sxx/1
  Transfer Function 1/3("TF ") -> Format Data  for Workspace/2(Sxy)
  Transfer Function 1/1(TF Mag) -> Sxy/1
  "Transfer Function "/3("TF ") -> Format Data  for Workspace/1(Syy)
  sampler2/1 -> Format Data  for Workspace/3(Swap)
  connections:
  To Port 1/RConn1 -- Directional Bridge 3/RConn1
  To Port 2/RConn1 -- Directional Bridge 1/RConn1

== system simpower_extensions_1/Ideal 1:N Transformer ==
  CCS : powerlib/Electrical Sources/Controlled Current Source  Description=source block  DialogController=POWERSYS.PowerSysDialog  SystemSampleTime=-1  Initialize=off  Source_Type=AC  Amplitude=0  Phase=0  Frequency=0  Measurements=None
      settings: AttributesFormatString=\n
  CM : powerlib/Measurements/Current Measurement  Tag=PoWeRsYsTeMmEaSuReMeNt  DialogController=POWERSYS.PowerSysDialog  SystemSampleTime=-1  PhasorSimulation=off  OutputType=Magnitude  PSBequivalent=0
  CVS : powerlib/Electrical Sources/Controlled Voltage Source  Description=source block  DialogController=POWERSYS.PowerSysDialog  SystemSampleTime=-1  Initialize=off  Source_Type=AC  Amplitude=0  Phase=0  Frequency=0  Measurements=None
      settings: AttributesFormatString=\n
  Gain : Gain  Gain=-N  ParameterDataType=sfix(16)  ParameterScaling=2^0  OutDataType=sfix(16)  OutScaling=2^0  SaturateOnIntegerOverflow=on  OutDataTypeStr=Inherit: Same as input  ParamDataTypeStr=Inherit: Same as input
  Gain1 : Gain  Gain=N  ParameterDataType=sfix(16)  ParameterScaling=2^0  OutDataType=sfix(16)  OutScaling=2^0  SaturateOnIntegerOverflow=on  OutDataTypeStr=Inherit: Same as input  ParamDataTypeStr=Inherit: Same as input
  VM : powerlib/Measurements/Voltage Measurement  Tag=PoWeRsYsTeMmEaSuReMeNt  DialogController=POWERSYS.PowerSysDialog  SystemSampleTime=-1  PhasorSimulation=off  OutputType=Magnitude  PSBequivalent=0
  P1 : PMIOPort  Tag=PMCPort  Port=1  Side=Left
  P2 : PMIOPort  Tag=PMCPort  Port=2  Side=Left
  S1 : PMIOPort  Tag=PMCPort  Port=3  Side=Right
  S2 : PMIOPort  Tag=PMCPort  Port=4  Side=Right
  wires:
  CM/1 -> Gain/1
  Gain/1 -> CCS/1
  Gain1/1 -> CVS/1
  VM/1 -> Gain1/1
  connections:
  CVS/LConn1 -- S2/RConn1
  CM/RConn1 -- CVS/RConn1
  CM/LConn1 -- S1/RConn1
  VM/LConn2 -- P2/RConn1 -- CCS/RConn1
  VM/LConn1 -- P1/RConn1 -- CCS/LConn1

== system simpower_extensions_1/NPN  Ebbers-Moll  ==
  note: Beta = 1/(1-AlphaF)
      | AlphaF=(Beta-1)/Beta
      | IEs*AlphaF=ICs*AlphaR
      |
      | Based on ....
      | http://ece-www.colorado.edu/~bart/book/book/chapter5/ch5_3.htm#5_3_3
      |
      | This is a 1st cut NON LINEAR model, not a final product!
  AlphaF : Gain  Gain=(Beta-1)/Beta  ParameterDataType=sfix(16)  ParameterScaling=2^0  OutDataType=sfix(16)  OutScaling=2^0
  AlphaF*If : powerlib/Electrical Sources/Controlled Current Source  Description=source block  DialogController=POWERSYS.PowerSysDialog  SystemSampleTime=-1  Initialize=off  Source_Type=AC  Amplitude=-0.025  Phase=0  Frequency=0  Measurements=None
      settings: AttributesFormatString=\n
  AlphaR : Gain  Gain=(IEs/ICs)*(Beta-1)/Beta  ParameterDataType=sfix(16)  ParameterScaling=2^0  OutDataType=sfix(16)  OutScaling=2^0
  AlphaR*Ir : powerlib/Electrical Sources/Controlled Current Source  Description=source block  DialogController=POWERSYS.PowerSysDialog  SystemSampleTime=-1  Initialize=off  Source_Type=AC  Amplitude=-0.025  Phase=0  Frequency=0  Measurements=None
      settings: AttributesFormatString=\n
  Base Emitter Junction : Subsystem  AncestorBlock=simcircuits_library_1/diode  mask{Is=IEs}
      mask prompts: Is "Saturation Current"
      mask Display: plot(-140,-140,150,140,2*[30,30,59,30,30,0]-75,(2*[71,50,72,92,71,71]-92),2*[59,59]-75,(2*[50,93]-92),[116,59]-16,(2*[71,71]-90));
  Cbc : powerlib/Elements/Parallel RLC Branch  DialogController=POWERSYS.PowerSysDialog  PhysicalDomain=powersysdomain  SubClassName=unknown  LeftPortType=p1  RightPortType=p1  LConnTagsString=a  RConnTagsString=__new0  BranchType=RLC  Resistance=inf  Inductance=inf  SetiL0=off  InitialCurrent=0  Capacitance=Cbc  Setx0=off  InitialVoltage=0  Measurements=None
  Cbe : powerlib/Elements/Parallel RLC Branch  DialogController=POWERSYS.PowerSysDialog  PhysicalDomain=powersysdomain  SubClassName=unknown  LeftPortType=p1  RightPortType=p1  LConnTagsString=a  RConnTagsString=__new0  BranchType=RLC  Resistance=inf  Inductance=inf  SetiL0=off  InitialCurrent=0  Capacitance=Cbe  Setx0=off  InitialVoltage=0  Measurements=None
  Collector Base Junction : Subsystem  AncestorBlock=simcircuits_library_1/diode  mask{Is=ICs}
      mask prompts: Is "Saturation Current"
      mask Display: plot(-140,-140,150,140,2*[30,30,59,30,30,0]-75,(2*[71,50,72,92,71,71]-92),2*[59,59]-75,(2*[50,93]-92),[116,59]-16,(2*[71,71]-90));
  Rbb : powerlib/Elements/Series RLC Branch  DialogController=POWERSYS.PowerSysDialog  PhysicalDomain=powersysdomain  SubClassName=unknown  LeftPortType=p1  RightPortType=p1  LConnTagsString=__new0  RConnTagsString=__new0  BranchType=R  Resistance=Rbb  Inductance=1.0  SetiL0=off  InitialCurrent=0  Capacitance=1.0  Setx0=off  InitialVoltage=0  Measurements=None
  Ro : powerlib/Elements/Parallel RLC Branch  DialogController=POWERSYS.PowerSysDialog  PhysicalDomain=powersysdomain  SubClassName=unknown  LeftPortType=p1  RightPortType=p1  LConnTagsString=a  RConnTagsString=__new0  BranchType=RLC  Resistance=Ro  Inductance=inf  SetiL0=off  InitialCurrent=0  Capacitance=0  Setx0=off  InitialVoltage=0  Measurements=None
  Base : PMIOPort  Port=1  Side=Left
  Collector : PMIOPort  Port=2  Side=Right
  Emitter : PMIOPort  Port=3  Side=Right
  wires:
  AlphaR/1 -> AlphaR*Ir/1
  Collector Base Junction/1(Idiode) -> AlphaR/1
  AlphaF/1 -> AlphaF*If/1
  Base Emitter Junction/1(Idiode) -> AlphaF/1  "If"
  connections:
  Rbb/LConn1 -- Base/RConn1
  Ro/RConn1 -- Collector Base Junction/RConn1 -- Cbc/LConn1 -- Collector/RConn1 -- AlphaF*If/LConn1
  Base Emitter Junction/RConn1 -- Ro/LConn1 -- Cbe/RConn1 -- Emitter/RConn1 -- AlphaR*Ir/LConn1
  Collector Base Junction/LConn1 -- AlphaR*Ir/RConn1 -- Cbc/RConn1 -- AlphaF*If/RConn1 -- Base Emitter Junction/LConn1 -- Cbe/LConn1 -- Rbb/RConn1

== system simpower_extensions_1/PNP Ebbers-Moll ==
  note: PNP
  note: Beta = 1/(1-AlphaF)
      | AlphaF=(Beta-1)/Beta
      | IEs*AlphaF=ICs*AlphaR
      |
      | Based on ....
      | http://ece-www.colorado.edu/~bart/book/book/chapter5/ch5_3.htm#5_3_3
      |
      | This is a 1st cut NON LINEAR model, not a final product!
  AlphaF : Gain  Gain=-(Beta-1)/Beta  ParameterDataType=sfix(16)  ParameterScaling=2^0  OutDataType=sfix(16)  OutScaling=2^0
  AlphaF*If : powerlib/Electrical Sources/Controlled Current Source  Description=source block  DialogController=POWERSYS.PowerSysDialog  SystemSampleTime=-1  Initialize=off  Source_Type=AC  Amplitude=-0.025  Phase=0  Frequency=0  Measurements=None
      settings: AttributesFormatString=\n
  AlphaR : Gain  Gain=-(IEs/ICs)*(Beta-1)/Beta  ParameterDataType=sfix(16)  ParameterScaling=2^0  OutDataType=sfix(16)  OutScaling=2^0
  AlphaR*Ir : powerlib/Electrical Sources/Controlled Current Source  Description=source block  DialogController=POWERSYS.PowerSysDialog  SystemSampleTime=-1  Initialize=off  Source_Type=AC  Amplitude=-0.025  Phase=0  Frequency=0  Measurements=None
      settings: AttributesFormatString=\n
  Base Emitter Junction : Subsystem  AncestorBlock=simcircuits_library_1/diode  mask{Is=IEs}
      mask prompts: Is "Saturation Current"
      mask Display: plot(-140,-140,150,140,2*[30,30,59,30,30,0]-75,(2*[71,50,72,92,71,71]-92),2*[59,59]-75,(2*[50,93]-92),[116,59]-16,(2*[71,71]-90));
  Cbc : powerlib/Elements/Parallel RLC Branch  DialogController=POWERSYS.PowerSysDialog  PhysicalDomain=powersysdomain  SubClassName=unknown  LeftPortType=p1  RightPortType=p1  LConnTagsString=a  RConnTagsString=__new0  BranchType=RLC  Resistance=inf  Inductance=inf  SetiL0=off  InitialCurrent=0  Capacitance=Cbc  Setx0=off  InitialVoltage=0  Measurements=None
  Cbe : powerlib/Elements/Parallel RLC Branch  DialogController=POWERSYS.PowerSysDialog  PhysicalDomain=powersysdomain  SubClassName=unknown  LeftPortType=p1  RightPortType=p1  LConnTagsString=a  RConnTagsString=__new0  BranchType=RLC  Resistance=inf  Inductance=inf  SetiL0=off  InitialCurrent=0  Capacitance=Cbe  Setx0=off  InitialVoltage=0  Measurements=None
  Collector Base Junction : Subsystem  AncestorBlock=simcircuits_library_1/diode  mask{Is=ICs}
      mask prompts: Is "Saturation Current"
      mask Display: plot(-140,-140,150,140,2*[30,30,59,30,30,0]-75,(2*[71,50,72,92,71,71]-92),2*[59,59]-75,(2*[50,93]-92),[116,59]-16,(2*[71,71]-90));
  Rbb : powerlib/Elements/Series RLC Branch  DialogController=POWERSYS.PowerSysDialog  PhysicalDomain=powersysdomain  SubClassName=unknown  LeftPortType=p1  RightPortType=p1  LConnTagsString=__new0  RConnTagsString=__new0  BranchType=R  Resistance=Rbb  Inductance=1.0  SetiL0=off  InitialCurrent=0  Capacitance=1.0  Setx0=off  InitialVoltage=0  Measurements=None
  Ro : powerlib/Elements/Parallel RLC Branch  DialogController=POWERSYS.PowerSysDialog  PhysicalDomain=powersysdomain  SubClassName=unknown  LeftPortType=p1  RightPortType=p1  LConnTagsString=a  RConnTagsString=__new0  BranchType=RLC  Resistance=Ro  Inductance=inf  SetiL0=off  InitialCurrent=0  Capacitance=0  Setx0=off  InitialVoltage=0  Measurements=None
  Base : PMIOPort  Port=1  Side=Left
  Emitter : PMIOPort  Port=2  Side=Right
  Collector : PMIOPort  Port=3  Side=Right
  wires:
  AlphaR/1 -> AlphaR*Ir/1
  Collector Base Junction/1(Idiode) -> AlphaR/1
  AlphaF/1 -> AlphaF*If/1
  Base Emitter Junction/1(Idiode) -> AlphaF/1  "If"
  connections:
  Rbb/LConn1 -- Base/RConn1
  Collector Base Junction/LConn1 -- Cbc/LConn1 -- Collector/RConn1 -- AlphaF*If/LConn1 -- Ro/RConn1
  Base Emitter Junction/LConn1 -- AlphaR*Ir/LConn1 -- Ro/LConn1 -- Cbe/RConn1 -- Emitter/RConn1
  Base Emitter Junction/RConn1 -- Cbc/RConn1 -- AlphaF*If/RConn1 -- Cbe/LConn1 -- Rbb/RConn1 -- AlphaR*Ir/RConn1 -- Collector Base Junction/RConn1

== system simpower_extensions_1/RF Spectum Analyzer (Image Reject) ==
  note: sine
  note: cosine
  Input Signal : Inport  OutDataType=sfix(16)  OutScaling=2^0
  Gain : Gain  Gain=1/sqrt(Zo)  ParameterDataType=fixdt(1, 16)  ParameterScaling=2^0  OutDataType=fixdt(1, 16)  OutScaling=2^0
  Real-Imag to Complex : RealImagToComplex
  Sine Wave1 : Sin  Amplitude=sqrt(2)  Bias=0  Frequency=2*pi*(Fc)  Phase=-pi/2  Samples=10  SampleTime=0  Offset=0
  Sine Wave2 : Sin  Amplitude=sqrt(2)  Bias=0  Frequency=2*pi*(Fc)  Phase=0  Samples=10  SampleTime=0  Offset=0
  Spectrum Scope : dspsnks4/Spectrum Scope  DialogController=dspdialog.SpectrumScope  DialogControllerArgs=DataTag34  SystemSampleTime=-1  ScopeProperties=on  Domain=Frequency  HorizSpan=1  UseBuffer=on  BufferSize=256  Overlap=64  inpFftLenInherit=off  FFTlength=128  numAvg=2  DisplayProperties=off  AxisGrid=on  Memory=off  FrameNumber=on  AxisLegend=off  AxisZoom=off  OpenScopeAtSimStart=on  OpenScopeImmediately=off  FigPos=[626 37 392 254]  AxisProperties=off  XUnits=Hertz  XRange=Two-sided ((-Fs/2...Fs/2])  XDisplay=0  InheritXIncr=on  XIncr=1.0  XLabel=Samples  XLimit=Auto  YUnits=dBm  XMax=1  XMin=0  YLabel=dBm  LineProperties=off  wintypeSpecScope=Hann  RsSpecScope=50  betaSpecScope=5  winsampSpecScope=Periodic  XAxisParamsVer=6.9
      settings: YMin=-70  YMax=30
  anti alias : dsparch4/Analog Filter Design  method=Elliptic  filttype=Lowpass  N=9  Wlo=BW*pi  Whi=80  Rp=1.2  Rs=100
  anti alias1 : dsparch4/Analog Filter Design  method=Elliptic  filttype=Lowpass  N=9  Wlo=BW*pi  Whi=80  Rp=1.2  Rs=100
  down convert : Product  OutDataType=sfix(16)  OutScaling=2^0  SaturateOnIntegerOverflow=on  InputSameDT=on  OutDataTypeStr=Inherit: Same as first input
  down convert1 : Product  OutDataType=sfix(16)  OutScaling=2^0  SaturateOnIntegerOverflow=on  InputSameDT=on  OutDataTypeStr=Inherit: Same as first input
  sampler (imag) : ZeroOrderHold  SampleTime=1/(1.28*BW)
  sampler (real) : ZeroOrderHold  SampleTime=1/(1.28*BW)
  wires:
  Gain/1 -> Spectrum Scope/1
  Real-Imag to Complex/1 -> Gain/1
  sampler (imag)/1 -> Real-Imag to Complex/2
  sampler (real)/1 -> Real-Imag to Complex/1
  down convert1/1 -> anti alias1/1
  anti alias1/1 -> sampler (imag)/1
  Sine Wave2/1 -> down convert1/2
  Sine Wave1/1 -> down convert/1
  anti alias/1 -> sampler (real)/1
  down convert/1 -> anti alias/1
  Input Signal/1 -> down convert1/1, down convert/2

== system simpower_extensions_1/Small Signal  Transistor Model ==
  -Gm : Gain  Gain=-gm  ParameterDataType=sfix(16)  ParameterScaling=2^0  OutDataType=sfix(16)  OutScaling=2^0  SaturateOnIntegerOverflow=on  OutDataTypeStr=Inherit: Same as input  ParamDataTypeStr=Inherit: Same as input
  -Gm*Vbe : powerlib/Electrical Sources/Controlled Current Source  Description=source block  DialogController=POWERSYS.PowerSysDialog  SystemSampleTime=-1  Initialize=off  Source_Type=AC  Amplitude=-0.025  Phase=0  Frequency=0  Measurements=None
      settings: AttributesFormatString=\n
  Rbb : powerlib/Elements/Series RLC Branch  DialogController=POWERSYS.PowerSysDialog  PhysicalDomain=powersysdomain  SubClassName=unknown  LeftPortType=p1  RightPortType=p1  LConnTagsString=__new0  RConnTagsString=__new0  BranchType=R  Resistance=Rbb  Inductance=1.0  SetiL0=off  InitialCurrent=0  Capacitance=1.0  Setx0=off  InitialVoltage=0  Measurements=None
  "Rbc, Cbc" : powerlib/Elements/Parallel RLC Branch  DialogController=POWERSYS.PowerSysDialog  PhysicalDomain=powersysdomain  SubClassName=unknown  LeftPortType=p1  RightPortType=p1  LConnTagsString=a  RConnTagsString=__new0  BranchType=RLC  Resistance=Rbc  Inductance=inf  SetiL0=off  InitialCurrent=0  Capacitance=Cbc  Setx0=off  InitialVoltage=0  Measurements=None
  "Rbe, Cbe" : powerlib/Elements/Parallel RLC Branch  DialogController=POWERSYS.PowerSysDialog  PhysicalDomain=powersysdomain  SubClassName=unknown  LeftPortType=p1  RightPortType=p1  LConnTagsString=a  RConnTagsString=__new0  BranchType=RLC  Resistance=Rbe  Inductance=inf  SetiL0=off  InitialCurrent=0  Capacitance=Cbe  Setx0=off  InitialVoltage=0  Measurements=None
  Vbe : powerlib/Measurements/Voltage Measurement  Tag=PoWeRsYsTeMmEaSuReMeNt  DialogController=POWERSYS.PowerSysDialog  SystemSampleTime=-1  PhasorSimulation=off  OutputType=Magnitude  PSBequivalent=0
  Base : PMIOPort  Port=1  Side=Left
  Collector : PMIOPort  Port=2  Side=Right
  Emitter : PMIOPort  Port=3  Side=Right
  wires:
  Vbe/1 -> -Gm/1
  -Gm/1 -> -Gm*Vbe/1
  connections:
  Collector/RConn1 -- -Gm*Vbe/RConn1 -- "Rbc, Cbc"/RConn1
  Vbe/LConn2 -- "Rbe, Cbe"/RConn1 -- Emitter/RConn1 -- -Gm*Vbe/LConn1
  "Rbc, Cbc"/LConn1 -- "Rbe, Cbe"/LConn1 -- Vbe/LConn1 -- Rbb/RConn1
  Base/RConn1 -- Rbb/LConn1

== system simpower_extensions_1/Spectrum ==
  Input Signal : Inport  OutDataType=sfix(16)  OutScaling=2^0
  Gain : Gain  Gain=1/sqrt(Zo)  ParameterDataType=fixdt(1, 16)  ParameterScaling=2^0  OutDataType=fixdt(1, 16)  OutScaling=2^0
  Spectrum Scope : dspsnks4/Spectrum Scope  DialogController=dspdialog.SpectrumScope  DialogControllerArgs=DataTag35  SystemSampleTime=-1  ScopeProperties=on  Domain=Frequency  HorizSpan=1  UseBuffer=on  BufferSize=512  Overlap=0  inpFftLenInherit=off  FFTlength=128  numAvg=1  DisplayProperties=off  AxisGrid=on  Memory=off  FrameNumber=on  AxisLegend=off  AxisZoom=off  OpenScopeAtSimStart=on  OpenScopeImmediately=off  FigPos=[575 32 408 280]  AxisProperties=off  XUnits=Hertz  XRange=One-sided ([0...Fs/2])  XDisplay=0  InheritXIncr=on  XIncr=1.0  XLabel=Samples  XLimit=Auto  YUnits=dBm  XMax=1  XMin=0  YLabel=dBm  LineProperties=off  wintypeSpecScope=Hann  RsSpecScope=50  betaSpecScope=5  winsampSpecScope=Periodic  XAxisParamsVer=6.9
      settings: YMin=-70  YMax=30
  anti alias : dsparch4/Analog Filter Design  method=Elliptic  filttype=Lowpass  N=8  Wlo=BW*2*pi  Whi=80  Rp=0.11  Rs=100
  sampler : ZeroOrderHold  SampleTime=1/(2.56*BW)
  wires:
  sampler/1 -> Gain/1
  anti alias/1 -> sampler/1
  Input Signal/1 -> anti alias/1
  Gain/1 -> Spectrum Scope/1

== system simpower_extensions_1/Varactor  (voltage variable capacitor) ==
  "C vs V " : Subsystem
  CVS : powerlib/Electrical Sources/Controlled Voltage Source  Description=source block  DialogController=POWERSYS.PowerSysDialog  SystemSampleTime=-1  Initialize=on  Source_Type=AC  Amplitude=0  Phase=0  Frequency=0  Measurements=None
      settings: AttributesFormatString=\n
  IM : powerlib/Measurements/Current Measurement  Tag=PoWeRsYsTeMmEaSuReMeNt  DialogController=POWERSYS.PowerSysDialog  SystemSampleTime=-1  PhasorSimulation=off  OutputType=Magnitude  PSBequivalent=0
  Integrator : Integrator
  Product : Product  Inputs=*/  OutDataType=sfix(16)  OutScaling=2^0  SaturateOnIntegerOverflow=on  OutDataTypeStr=Inherit: Same as first input
  VM : powerlib/Measurements/Voltage Measurement  Tag=PoWeRsYsTeMmEaSuReMeNt  DialogController=POWERSYS.PowerSysDialog  SystemSampleTime=-1  PhasorSimulation=off  OutputType=Magnitude  PSBequivalent=0
  t1 : PMIOPort  Tag=PMCPort  Port=1  Side=Left
  "t2 " : PMIOPort  Tag=PMCPort  Port=2  Side=Right
  C : Outport  OutDataType=sfix(16)  OutScaling=2^0
  wires:
  "C vs V "/1(C) -> C/1, Product/2
  IM/1 -> Product/1
  VM/1 -> "C vs V "/1("Vr ")
  Product/1 -> Integrator/1
  Integrator/1 -> CVS/1
  connections:
  VM/LConn2 -- CVS/LConn1 -- "t2 "/RConn1
  IM/RConn1 -- CVS/RConn1
  IM/LConn1 -- VM/LConn1 -- t1/RConn1

== system simpower_extensions_1/Variable C ==
  C : Inport  OutDataType=sfix(16)  OutScaling=2^0
  CVS : powerlib/Electrical Sources/Controlled Voltage Source  Description=source block  DialogController=POWERSYS.PowerSysDialog  SystemSampleTime=-1  Initialize=off  Source_Type=AC  Amplitude=0  Phase=0  Frequency=0  Measurements=None
      settings: AttributesFormatString=\n
  IM : powerlib/Measurements/Current Measurement  Tag=PoWeRsYsTeMmEaSuReMeNt  DialogController=POWERSYS.PowerSysDialog  SystemSampleTime=-1  PhasorSimulation=off  OutputType=Magnitude  PSBequivalent=0
  Integrator : Integrator
  Product : Product  Inputs=*/  OutDataType=sfix(16)  OutScaling=2^0  SaturateOnIntegerOverflow=on  OutDataTypeStr=Inherit: Same as first input
  Cb : PMIOPort  Tag=PMCPort  Port=1  Side=Right
  Ca : PMIOPort  Tag=PMCPort  Port=2  Side=Left
  wires:
  C/1 -> Product/2
  IM/1 -> Product/1
  Product/1 -> Integrator/1
  Integrator/1 -> CVS/1
  connections:
  IM/LConn1 -- Ca/RConn1
  IM/RConn1 -- CVS/RConn1
  CVS/LConn1 -- Cb/RConn1

== system simpower_extensions_1/Variable L ==
  L : Inport  OutDataType=sfix(16)  OutScaling=2^0
  CCS1 : powerlib/Electrical Sources/Controlled Current Source  Description=source block  DialogController=POWERSYS.PowerSysDialog  SystemSampleTime=-1  Initialize=off  Source_Type=AC  Amplitude=0  Phase=0  Frequency=0  Measurements=None
      settings: AttributesFormatString=\n
  Divide : Product  Inputs=*/  OutDataType=sfix(16)  OutScaling=2^-10
  Int 1 : Integrator
  Voltage Measurement : powerlib/Measurements/Voltage Measurement  DialogController=POWERSYS.PowerSysDialog  SystemSampleTime=-1  PhasorSimulation=off  OutputType=Complex  PSBequivalent=0
  La : PMIOPort  Tag=PMCPort  Port=1  Side=Left
  Lb : PMIOPort  Tag=PMCPort  Port=2  Side=Right
  wires:
  L/1 -> Divide/2
  Int 1/1 -> Divide/1
  Divide/1 -> CCS1/1
  Voltage Measurement/1 -> Int 1/1
  connections:
  Voltage Measurement/LConn2 -- Lb/RConn1 -- CCS1/RConn1
  Voltage Measurement/LConn1 -- CCS1/LConn1 -- La/RConn1

== system simpower_extensions_1/Variable R ==
  R : Inport  OutDataType=sfix(16)  OutScaling=2^0
  CVS : powerlib/Electrical Sources/Controlled Voltage Source  Description=source block  DialogController=POWERSYS.PowerSysDialog  SystemSampleTime=-1  Initialize=off  Source_Type=AC  Amplitude=0  Phase=0  Frequency=0  Measurements=None
      settings: AttributesFormatString=\n
  IM : powerlib/Measurements/Current Measurement  Tag=PoWeRsYsTeMmEaSuReMeNt  DialogController=POWERSYS.PowerSysDialog  SystemSampleTime=-1  PhasorSimulation=off  OutputType=Magnitude  PSBequivalent=0
  Product : Product  Inputs=**  OutDataType=sfix(16)  OutScaling=2^0  SaturateOnIntegerOverflow=on  OutDataTypeStr=Inherit: Same as first input
  Rb : PMIOPort  Tag=PMCPort  Port=1  Side=Right
  Ra : PMIOPort  Tag=PMCPort  Port=2  Side=Left
  wires:
  R/1 -> Product/2
  IM/1 -> Product/1
  Product/1 -> CVS/1
  connections:
  IM/LConn1 -- Ra/RConn1
  IM/RConn1 -- CVS/RConn1
  CVS/LConn1 -- Rb/RConn1

== system simpower_extensions_1/activef ==

== system simpower_extensions_1/bpf ==
  Gain : Gain  ParameterDataType=sfix(16)  ParameterScaling=2^0  OutDataType=sfix(16)  OutScaling=2^0  SaturateOnIntegerOverflow=on  OutDataTypeStr=Inherit: Same as input  ParamDataTypeStr=Inherit: Same as input

== system simpower_extensions_1/bpf1 ==

== system simpower_extensions_1/bpf2 ==

== system simpower_extensions_1/bpf3 ==

== system simpower_extensions_1/bpf4 ==

== system simpower_extensions_1/bpf5 ==
  Gain : Gain  ParameterDataType=sfix(16)  ParameterScaling=2^0  OutDataType=sfix(16)  OutScaling=2^0  SaturateOnIntegerOverflow=on  OutDataTypeStr=Inherit: Same as input  ParamDataTypeStr=Inherit: Same as input

== system simpower_extensions_1/bpf6 ==
  Gain : Gain  ParameterDataType=sfix(16)  ParameterScaling=2^0  OutDataType=sfix(16)  OutScaling=2^0  SaturateOnIntegerOverflow=on  OutDataTypeStr=Inherit: Same as input  ParamDataTypeStr=Inherit: Same as input

== system simpower_extensions_1/bpf7 ==

== system simpower_extensions_1/bpf9 ==
  Gain : Gain  ParameterDataType=sfix(16)  ParameterScaling=2^0  OutDataType=sfix(16)  OutScaling=2^0  SaturateOnIntegerOverflow=on  OutDataTypeStr=Inherit: Same as input  ParamDataTypeStr=Inherit: Same as input

== system simpower_extensions_1/ce ==

== system simpower_extensions_1/cscd ==

== system simpower_extensions_1/cscd1 ==

== system simpower_extensions_1/cscd10 ==

== system simpower_extensions_1/cscd11 ==

== system simpower_extensions_1/cscd12 ==

== system simpower_extensions_1/cscd13 ==

== system simpower_extensions_1/cscd14 ==

== system simpower_extensions_1/cscd15 ==

== system simpower_extensions_1/cscd2 ==

== system simpower_extensions_1/cscd3 ==

== system simpower_extensions_1/cscd4 ==

== system simpower_extensions_1/cscd5 ==

== system simpower_extensions_1/cscd6 ==

== system simpower_extensions_1/cscd7 ==

== system simpower_extensions_1/cscd8 ==

== system simpower_extensions_1/cscd9 ==
